simulink model "L4_3_param_sweep"  (R2025b)
settings: Solver=VariableStepAuto  StartTime=0.0  StopTime=10  MaxStep=0.05  RelTol=1e-3
undefined symbols (not defined in the file): Kp_val
settings Model: Creator=kimsteph  LastModifiedBy=kimsteph

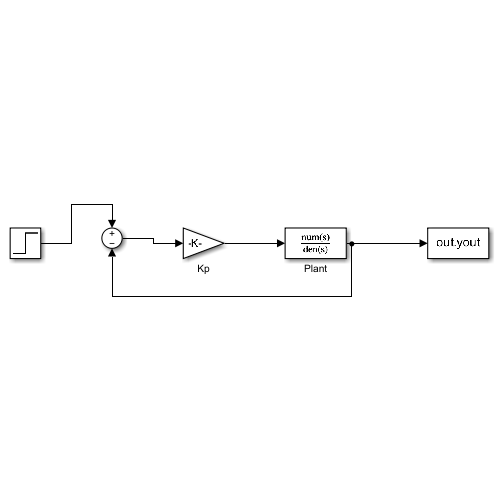
[thumbnail: Simulink's stored preview of the top-level diagram]
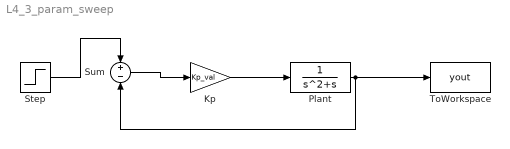
== system L4_3_param_sweep ==
  Kp : Gain  Gain=Kp_val
  Plant : TransferFcn  Denominator=[1 1 0]
  Step : Step  Time=0  SampleTime=0
  Sum : Sum  Inputs=+-
  ToWorkspace : ToWorkspace  VariableName=yout  SaveFormat=Timeseries  SampleTime=-1
  wires:
  Step/1 -> Sum/1
  Sum/1 -> Kp/1
  Kp/1 -> Plant/1
  Plant/1 -> ToWorkspace/1, Sum/2
